simulink model "QuadCopterwhole"  (R2014b)
settings: Solver=ode23t  StartTime=0.0  StopTime=100  FixedStep=0.001  RelTol=1e-3  AbsTol=1e-4
InitFcn:
  | load SimpleDroneData
values from neighbouring files (symbols this model uses):
  m_indoorHull = 0.458    [QuadCopterParameters_m.m]
  motorCoeffs = [0.00010909388854752541 0.0075590948720063037 0.09060950915942291                 ]    [QuadCopterParameters_m.m]
libraries: simulink x2, vrlib x2, aerolibobsolete x1, aerolibtransform2 x1
settings Model: Creator=rruff  LastModifiedBy=Ehang
settings DataIOCC: SignalLoggingSaveFormat=ModelDataLogs  SaveOutput=off  SaveTime=off
settings OptimizationCC: InlineParams=on  ExpressionDepthLimit=2147483647  LifeSpan=1
settings DebuggingCC: UnderspecifiedInitializationDetection=Classic  MergeDetectMultiDrivingBlocksExec=none  SolverPrmCheckMsg=none  MultiTaskDSMMsg=warning  MultiTaskCondExecSysMsg=none  FcnCallInpInsideContextMsg=EnableAllAsWarning  StateNameClashWarn=warning
settings HardwareCC: ProdBitPerInt=16  ProdBitPerPointer=8  ProdIntDivRoundTo=Zero  ProdEndianess=LittleEndian  ProdWordSize=8  ProdHWDeviceType=Atmel->AVR
settings RTWCC: IncludeERTFirstTime=on
settings SimscapeCC: SelectedTab=SimMechanics2G
settings SimMechanicsCC: VisOnUpdateDiagram=on  VisDuringSimulation=on  FramesToBeSkipped=10  AnimationDelay=0  LastVizWinPosition=[1022 659 560 420]  CamPosition=[10.2752;-3.21889;-2.95529;]  CamTarget=[0;-2.23517e-09;-0.0242675;]  CamUpVector=[-0.23308;0.133123;-0.963303;]  CamHeight=0.224542  VisBackgroundColor=[0.9;0.9;0.95;]  DefaultBodyColor=[1;0;0;]
settings ExplorerConfigSet: SimMechanicsOpenEditorOnUpdate=off

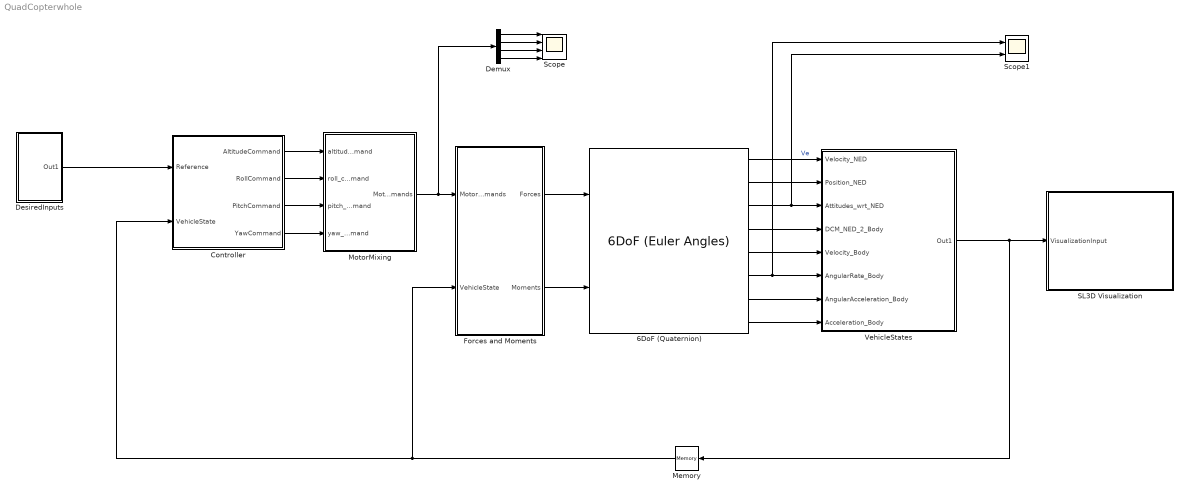
== system QuadCopterwhole ==
  6DoF (Quaternion) : aerolibobsolete/6DoF (Euler Angles)  units=Metric (MKS)  mtype=Fixed  rep=Quaternion  xme_0=[0 0 0]  Vm_0=[0 0 0]  eul_0=[0 0 0]  pm_0=[0 0 0]  mass_0=Mass  mass_e=0  mass_f=0  inertia=MomentInertiaTensor  inertia_e=eye(3)  inertia_f=eye(3)  k_quat=1.0
  Controller : Subsystem
  Demux : Demux
  DesiredInputs : Subsystem
  Forces and Moments : Subsystem  TreatAsAtomicUnit=on
  Memory : Memory
  MotorMixing : Subsystem
  SL3D Visualization : Subsystem
  Scope : Scope  NumInputPorts=4
      settings: YMin=-5~-5~-5~-5  YMax=5~5~5~5
  Scope1 : Scope  NumInputPorts=2
      settings: YMin=-5~-5  YMax=5~5  SaveName=ScopeData5
  VehicleStates : Subsystem
  wires:
  Forces and Moments/1(Forces) -> 6DoF (Quaternion)/1
  Forces and Moments/2(Moments) -> 6DoF (Quaternion)/2
  6DoF (Quaternion)/6 -> Scope1/1, VehicleStates/6(AngularRate_Body)
  6DoF (Quaternion)/8 -> VehicleStates/8(Acceleration_Body)
  6DoF (Quaternion)/4 -> VehicleStates/4(DCM_NED_2_Body)
  6DoF (Quaternion)/5 -> VehicleStates/5(Velocity_Body)
  6DoF (Quaternion)/7 -> VehicleStates/7(AngularAcceleration_Body)
  6DoF (Quaternion)/3 -> Scope1/2, VehicleStates/3(Attitudes_wrt_NED)
  6DoF (Quaternion)/2 -> VehicleStates/2(Position_NED)
  6DoF (Quaternion)/1 -> VehicleStates/1(Velocity_NED)  "Ve"
  Controller/1(AltitudeCommand) -> MotorMixing/1(altitude_command)
  Controller/2(RollCommand) -> MotorMixing/2(roll_command)
  Controller/3(PitchCommand) -> MotorMixing/3(pitch_command)
  MotorMixing/1(MotorCommands) -> Demux/1, Forces and Moments/1(MotorCommands)
  Controller/4(YawCommand) -> MotorMixing/4(yaw_command)
  Memory/1 -> Controller/2(VehicleState), Forces and Moments/2(VehicleState)
  VehicleStates/1(Out1) -> SL3D Visualization/1(VisualizationInput), Memory/1
  DesiredInputs/1(Out1) -> Controller/1(Reference)
  Demux/2 -> Scope/2
  Demux/1 -> Scope/1
  Demux/3 -> Scope/3
  Demux/4 -> Scope/4

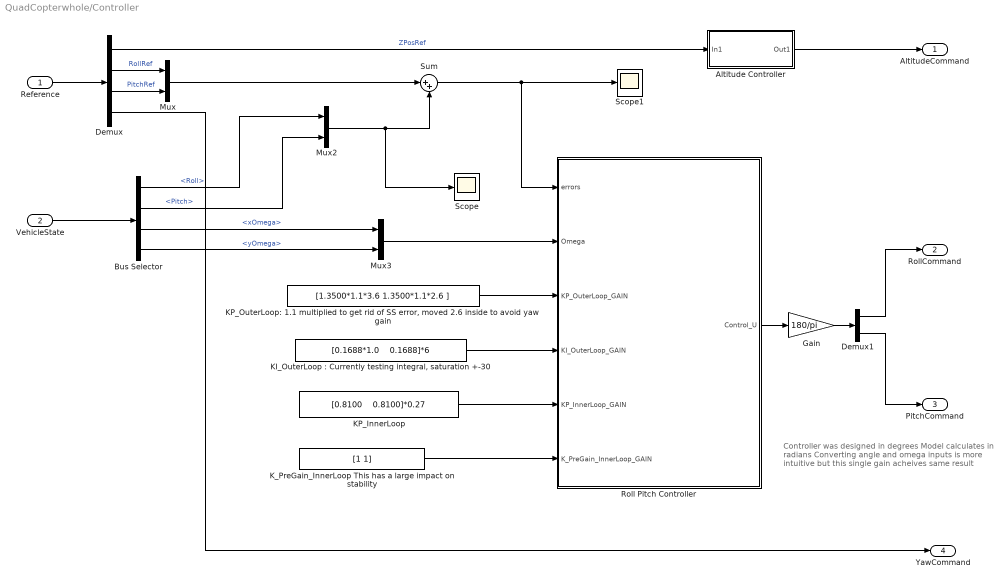
== system QuadCopterwhole/Controller ==
  note: Controller was designed in degrees
      | Model calculates in radians
      | Converting angle and omega inputs is more
      | intuitive but this single gain acheives same result
  Reference : Inport
  VehicleState : Inport  Port=2
  Altitude Controller : Subsystem
  Bus Selector : BusSelector  OutputSignals=NEDState.Attitude.Roll,NEDState.Attitude.Pitch,BodyState.AngularRate.xOmega,BodyState.AngularRate.yOmega
  Demux : Demux
  Demux1 : Demux  Outputs=2
  Gain : Gain  Gain=180/pi
  "KI_OuterLoop : Currently testing integral, saturation +-30" : Constant  Value="[0.1688*1.0    0.1688]*6"
  KP_InnerLoop : Constant  Value="[0.8100    0.8100]*0.27"
  "KP_OuterLoop: 1.1 multiplied to get rid of SS error, moved 2.6 inside to avoid yaw gain" : Constant  Value=[1.3500*1.1*3.6 1.3500*1.1*2.6 ]
  K_PreGain_InnerLoop This has a large impact on stability : Constant  Value=[1 1]
  Mux : Mux  Inputs=2
  Mux2 : Mux  Inputs=2
  Mux3 : Mux  Inputs=2
  Roll Pitch Controller : Subsystem  TreatAsAtomicUnit=on
  Scope : Scope
      settings: SaveName=ScopeData3
  Scope1 : Scope
      settings: SaveName=ScopeData11
  Sum : Sum  Inputs=|++
  AltitudeCommand : Outport
  RollCommand : Outport  Port=2
  PitchCommand : Outport  Port=3
  YawCommand : Outport  Port=4
  wires:
  Reference/1 -> Demux/1
  VehicleState/1 -> Bus Selector/1
  Demux/1 -> Altitude Controller/1(In1)  "ZPosRef"
  Demux/3 -> Mux/2  "PitchRef"
  Demux/2 -> Mux/1  "RollRef"
  Mux/1 -> Sum/1
  Mux2/1 -> Scope/1, Sum/2
  Sum/1 -> Scope1/1, Roll Pitch Controller/1(errors)
  Bus Selector/1 -> Mux2/1  "<Roll>"
  Bus Selector/2 -> Mux2/2  "<Pitch>"
  Bus Selector/3 -> Mux3/1  "<xOmega>"
  Bus Selector/4 -> Mux3/2  "<yOmega>"
  Mux3/1 -> Roll Pitch Controller/2(Omega)
  "KP_OuterLoop: 1.1 multiplied to get rid of SS error, moved 2.6 inside to avoid yaw gain"/1 -> Roll Pitch Controller/3(KP_OuterLoop_GAIN)
  K_PreGain_InnerLoop This has a large impact on stability/1 -> Roll Pitch Controller/6(K_PreGain_InnerLoop_GAIN)
  KP_InnerLoop/1 -> Roll Pitch Controller/5(KP_InnerLoop_GAIN)
  "KI_OuterLoop : Currently testing integral, saturation +-30"/1 -> Roll Pitch Controller/4(KI_OuterLoop_GAIN)
  Roll Pitch Controller/1(Control_U) -> Gain/1
  Demux1/1 -> RollCommand/1
  Demux1/2 -> PitchCommand/1
  Demux/4 -> YawCommand/1
  Gain/1 -> Demux1/1
  Altitude Controller/1(Out1) -> AltitudeCommand/1

== system QuadCopterwhole/DesiredInputs ==
  Mux : Mux
  Step : Step  Time=3  After=-1  SampleTime=0
  Step1 : Step  Time=2  After=0  SampleTime=0
  Step2 : Step  Time=5  After=0  SampleTime=0
  Step3 : Step  Time=5  After=0  SampleTime=0
  Out1 : Outport
  wires:
  Step1/1 -> Mux/2  "RollRef"
  Step/1 -> Mux/1  "ZPosRef"
  Step2/1 -> Mux/3  "PitchRef"
  Mux/1 -> Out1/1  "Reference"
  Step3/1 -> Mux/4  "YawRef"

== system QuadCopterwhole/Forces and Moments ==
  MotorCommands : Inport
  VehicleState : Inport  Port=2
  Applied Force Calculation : Subsystem
  Applied torque Calculation1 : Subsystem
  Display : Display
  Gravity Force Calculation : Subsystem
  Motor Forces and Torques : Subsystem
  Scope : Scope
      settings: SaveName=ScopeData4
  Forces : Outport
  Moments : Outport  Port=2
  wires:
  Motor Forces and Torques/1(Motor Forces) -> Applied torque Calculation1/1(Motor Forces), Applied Force Calculation/2(Motor Forces)
  Applied Force Calculation/1(External Forces) -> Forces/1
  Motor Forces and Torques/2(Motor Torques) -> Applied torque Calculation1/2(Motor Torques)
  Applied torque Calculation1/1(External Torques) -> Display/1, Moments/1
  MotorCommands/1 -> Motor Forces and Torques/1(Motor Commands)
  VehicleState/1 -> Gravity Force Calculation/1(posinfo)
  Gravity Force Calculation/1(gravity force) -> Scope/1, Applied Force Calculation/1(gravity force)

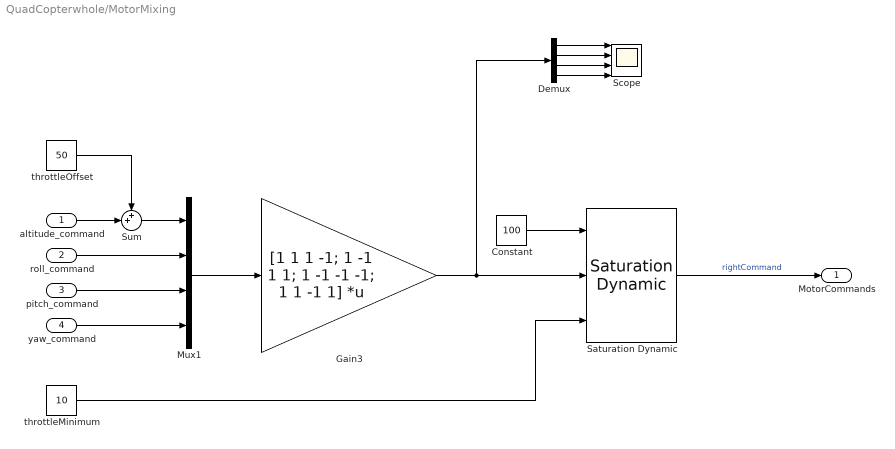
== system QuadCopterwhole/MotorMixing ==
  altitude_command : Inport
  roll_command : Inport  Port=2
  pitch_command : Inport  Port=3
  yaw_command : Inport  Port=4
  Constant : Constant  Value=100
  Demux : Demux
  Gain3 : Gain  Gain=[1 1 1 -1; 1 -1 1 1; 1 -1 -1 -1; 1 1 -1 1]  Multiplication=Matrix(K*u)  ParamDataTypeStr=int16
  Mux1 : Mux
  Saturation Dynamic : simulink/Discontinuities/Saturation Dynamic  OutMin=[]  OutMax=[]  OutDataTypeStr=Inherit: Same as second input  OutDataType=fixdt(1, 16)  OutScaling=2^-10  DoSatur=off
  Scope : Scope  NumInputPorts=4
      settings: TimeRange=100  YMin=-5~-5~-5~-5  YMax=5~5~5~5  SaveName=ScopeData2
  Sum : Sum  Inputs=++|
  throttleMinimum : Constant  Value=10
  throttleOffset : Constant  Value=50
  MotorCommands : Outport
  wires:
  yaw_command/1 -> Mux1/4
  pitch_command/1 -> Mux1/3
  roll_command/1 -> Mux1/2
  Mux1/1 -> Gain3/1
  altitude_command/1 -> Sum/2
  Sum/1 -> Mux1/1
  throttleOffset/1 -> Sum/1
  throttleMinimum/1 -> Saturation Dynamic/3
  Constant/1 -> Saturation Dynamic/1
  Saturation Dynamic/1 -> MotorCommands/1  "rightCommand"
  Gain3/1 -> Demux/1, Saturation Dynamic/2
  Demux/2 -> Scope/2
  Demux/1 -> Scope/1
  Demux/3 -> Scope/3
  Demux/4 -> Scope/4

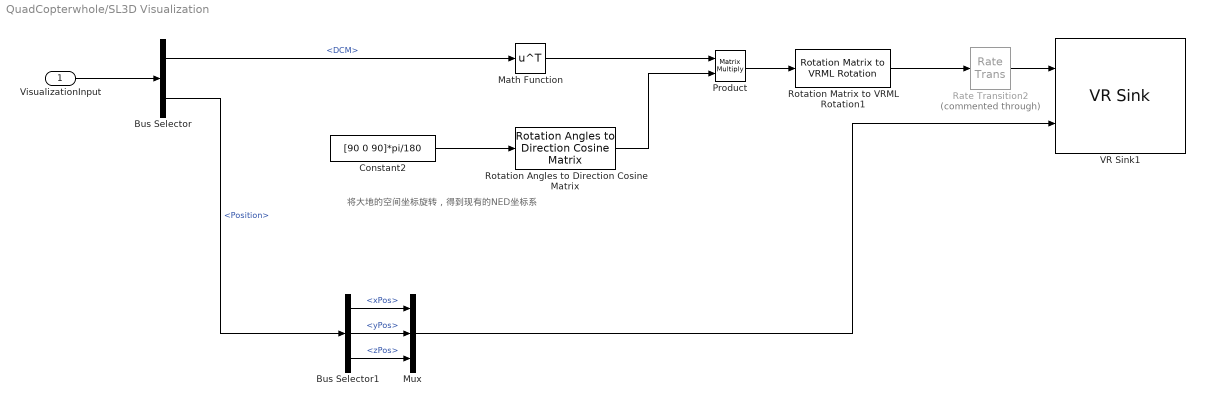
== system QuadCopterwhole/SL3D Visualization ==
  note: 将大地的空间坐标旋转，得到现有的NED坐标系
  VisualizationInput : Inport
  Bus Selector : BusSelector  OutputSignals=NEDState.Attitude.DCM,NEDState.Position
  Bus Selector1 : BusSelector  OutputSignals=xPos,yPos,zPos
  Constant2 : Constant  Value=[90 0 90]*pi/180
  Math Function : Math  Operator=transpose  SaturateOnIntegerOverflow=on
  Mux : Mux  Inputs=3
  Product : Product  Multiplication=Matrix(*)
  Rate Transition2 : RateTransition  Commented=through
  Rotation Angles to Direction Cosine Matrix : aerolibtransform2/Rotation Angles to Direction Cosine Matrix  rotationOrder=XYZ
  Rotation Matrix to VRML Rotation1 : vrlib/Utilities/Rotation Matrix to VRML Rotation  maxzero=1e-12
  VR Sink1 : vrlib/VR Sink  InstantiateOnLoad=on  SampleTime=-1  ViewEnable=on  RemoteChange=off  RemoteView=off  FieldsWritten=Drone.rotation.4.1.1.double#Drone.translation.3.1.1.double  WorldFileName=myDrone3.wrl  AutoView=off  VideoDimensions=[]  AllowVariableSize=off
  wires:
  VisualizationInput/1 -> Bus Selector/1
  Rotation Matrix to VRML Rotation1/1 -> Rate Transition2/1
  Rate Transition2/1 -> VR Sink1/1
  Bus Selector/2 -> Bus Selector1/1  "<Position>"
  Mux/1 -> VR Sink1/2
  Constant2/1 -> Rotation Angles to Direction Cosine Matrix/1
  Rotation Angles to Direction Cosine Matrix/1 -> Product/2
  Math Function/1 -> Product/1
  Product/1 -> Rotation Matrix to VRML Rotation1/1
  Bus Selector/1 -> Math Function/1  "<DCM>"
  Bus Selector1/1 -> Mux/1  "<xPos>"
  Bus Selector1/2 -> Mux/2  "<yPos>"
  Bus Selector1/3 -> Mux/3  "<zPos>"

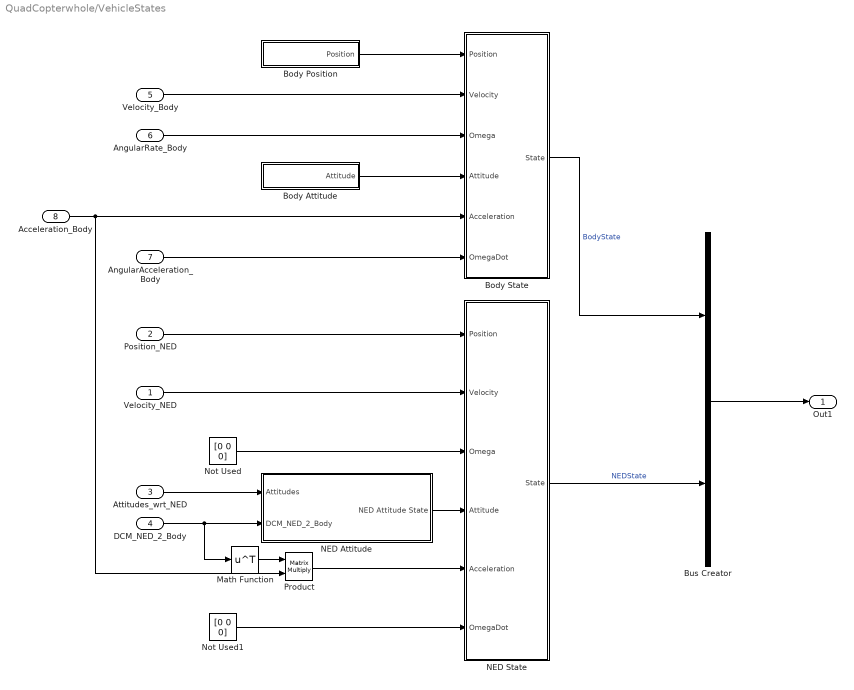
== system QuadCopterwhole/VehicleStates ==
  Velocity_NED : Inport
  Position_NED : Inport  Port=2
  Attitudes_wrt_NED : Inport  Port=3
  DCM_NED_2_Body : Inport  Port=4
  Velocity_Body : Inport  Port=5
  AngularRate_Body : Inport  Port=6
  AngularAcceleration_Body : Inport  Port=7
  Acceleration_Body : Inport  Port=8
  Body Attitude : Subsystem
  Body Position : Subsystem
  Body State : Subsystem
  Bus Creator : BusCreator  Inputs=2  OutDataTypeStr=Bus: VehicleStates  NonVirtualBus=on
  Math Function : Math  Operator=transpose  SaturateOnIntegerOverflow=on
  NED Attitude : Subsystem
  NED State : Subsystem
  Not Used : Constant  Value=[0 0 0]
  Not Used1 : Constant  Value=[0 0 0]
  Product : Product  Multiplication=Matrix(*)
  Out1 : Outport
  wires:
  Bus Creator/1 -> Out1/1
  Velocity_NED/1 -> NED State/2(Velocity)
  NED Attitude/1(NED Attitude State) -> NED State/4(Attitude)
  Position_NED/1 -> NED State/1(Position)
  Attitudes_wrt_NED/1 -> NED Attitude/1(Attitudes)
  NED State/1(State) -> Bus Creator/2  "NEDState"
  Body State/1(State) -> Bus Creator/1  "BodyState"
  Body Attitude/1(Attitude) -> Body State/4(Attitude)
  DCM_NED_2_Body/1 -> Math Function/1, NED Attitude/2(DCM_NED_2_Body)
  Acceleration_Body/1 -> Product/2, Body State/5(Acceleration)
  AngularAcceleration_Body/1 -> Body State/6(OmegaDot)
  Velocity_Body/1 -> Body State/2(Velocity)
  Body Position/1(Position) -> Body State/1(Position)
  AngularRate_Body/1 -> Body State/3(Omega)
  Not Used/1 -> NED State/3(Omega)
  Not Used1/1 -> NED State/6(OmegaDot)
  Product/1 -> NED State/5(Acceleration)
  Math Function/1 -> Product/1

== system QuadCopterwhole/Controller/Altitude Controller ==
  In1 : Inport
  Out1 : Outport
  wires:
  In1/1 -> Out1/1

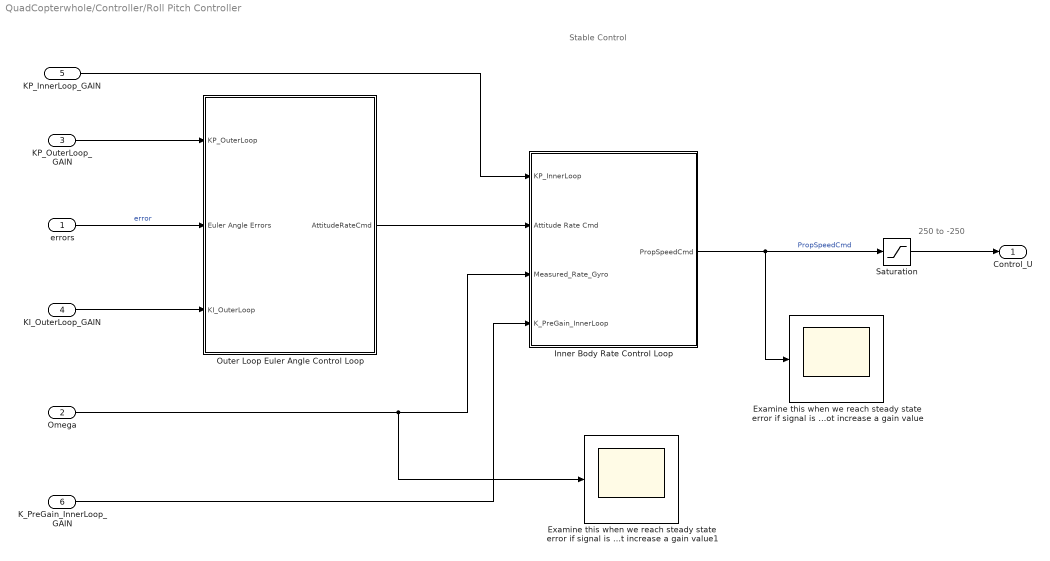
== system QuadCopterwhole/Controller/Roll Pitch Controller ==
  note: 250 to -250
  note: Stable Control
  errors : Inport
  Omega : Inport  Port=2
  KP_OuterLoop_GAIN : Inport  Port=3
  KI_OuterLoop_GAIN : Inport  Port=4
  KP_InnerLoop_GAIN : Inport  Port=5
  K_PreGain_InnerLoop_GAIN : Inport  Port=6
  Examine this when we reach steady state error if signal is abs(0)<1 then we need ot increase a gain value : Scope
      settings: YMin=-6  YMax=4  SaveName=ScopeData7
  Examine this when we reach steady state error if signal is abs(0)<1 then we need ot increase a gain value1 : Scope
      settings: YMin=-3.62958e-15  YMax=40
  Inner Body Rate Control Loop : Subsystem
  Outer Loop Euler Angle Control Loop : Subsystem
  Saturation : Saturate  UpperLimit=250  LowerLimit=-250  OutDataTypeStr=Inherit: Inherit via back propagation
      settings: AttributesFormatString=%<LowerLimit>\nto\n%<UpperLimit>
  Control_U : Outport
  wires:
  Saturation/1 -> Control_U/1
  KP_InnerLoop_GAIN/1 -> Inner Body Rate Control Loop/1(KP_InnerLoop)
  Omega/1 -> Examine this when we reach steady state error if signal is abs(0)<1 then we need ot increase a gain value1/1, Inner Body Rate Control Loop/3(Measured_Rate_Gyro)
  K_PreGain_InnerLoop_GAIN/1 -> Inner Body Rate Control Loop/4(K_PreGain_InnerLoop)
  Inner Body Rate Control Loop/1(PropSpeedCmd) -> Saturation/1, Examine this when we reach steady state error if signal is abs(0)<1 then we need ot increase a gain value/1  "PropSpeedCmd"
  KP_OuterLoop_GAIN/1 -> Outer Loop Euler Angle Control Loop/1(KP_OuterLoop)
  errors/1 -> Outer Loop Euler Angle Control Loop/2(Euler Angle Errors)  "error"
  KI_OuterLoop_GAIN/1 -> Outer Loop Euler Angle Control Loop/3(KI_OuterLoop)
  Outer Loop Euler Angle Control Loop/1(AttitudeRateCmd) -> Inner Body Rate Control Loop/2(Attitude Rate Cmd)

== system QuadCopterwhole/Forces and Moments/Applied Force Calculation ==
  gravity force : Inport
  Motor Forces : Inport  Port=2
  Add : Sum  Inputs=+
  Add1 : Sum
  Constant : Constant  Value=[0 0]
  Mux : Mux  Inputs=2
  External Forces : Outport
  wires:
  Add/1 -> Mux/2  "Vertical Thrust"
  Constant/1 -> Mux/1
  Add1/1 -> External Forces/1
  Motor Forces/1 -> Add/1
  Mux/1 -> Add1/2  "Motor Thrust"
  gravity force/1 -> Add1/1

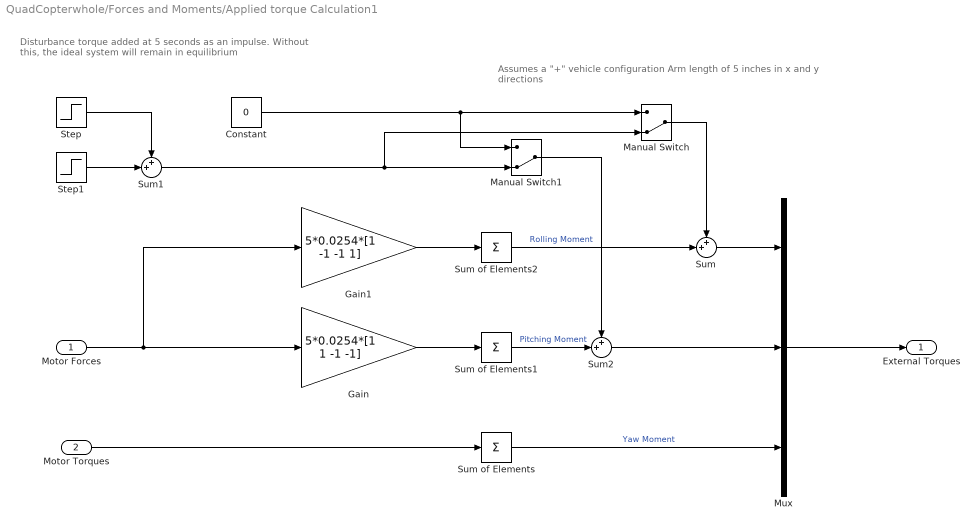
== system QuadCopterwhole/Forces and Moments/Applied torque Calculation1 ==
  note: Disturbance torque added at 5 seconds as an impulse.
      | Without this, the ideal system will remain in equilibrium
  note: Assumes a "+" vehicle configuration
      | Arm length of 5 inches in x and y directions
  Motor Forces : Inport
  Motor Torques : Inport  Port=2
  Constant : Constant  Value=0
  Gain : Gain  Gain=5*0.0254*[1 1 -1 -1]
  Gain1 : Gain  Gain=5*0.0254*[1 -1 -1 1]
  Manual Switch : ManualSwitch  CurrentSetting=0
  Manual Switch1 : ManualSwitch  CurrentSetting=0
  Mux : Mux  Inputs=3
  Step : Step  Time=5  SampleTime=0
  Step1 : Step  Time=5.01  After=-1  SampleTime=0
  Sum : Sum  Inputs=++|
  Sum of Elements : Sum  Inputs=+
  Sum of Elements1 : Sum  Inputs=+
  Sum of Elements2 : Sum  Inputs=+
  Sum1 : Sum  Inputs=++|
  Sum2 : Sum  Inputs=++|
  External Torques : Outport
  wires:
  Motor Torques/1 -> Sum of Elements/1
  Sum of Elements/1 -> Mux/3  "Yaw Moment"
  Motor Forces/1 -> Gain/1, Gain1/1
  Gain/1 -> Sum of Elements1/1
  Gain1/1 -> Sum of Elements2/1
  Mux/1 -> External Torques/1
  Sum/1 -> Mux/1
  Sum of Elements2/1 -> Sum/2  "Rolling Moment"
  Step1/1 -> Sum1/2
  Step/1 -> Sum1/1
  Sum2/1 -> Mux/2
  Sum of Elements1/1 -> Sum2/2  "Pitching Moment"
  Constant/1 -> Manual Switch1/1, Manual Switch/1
  Manual Switch/1 -> Sum/1
  Manual Switch1/1 -> Sum2/1
  Sum1/1 -> Manual Switch/2, Manual Switch1/2

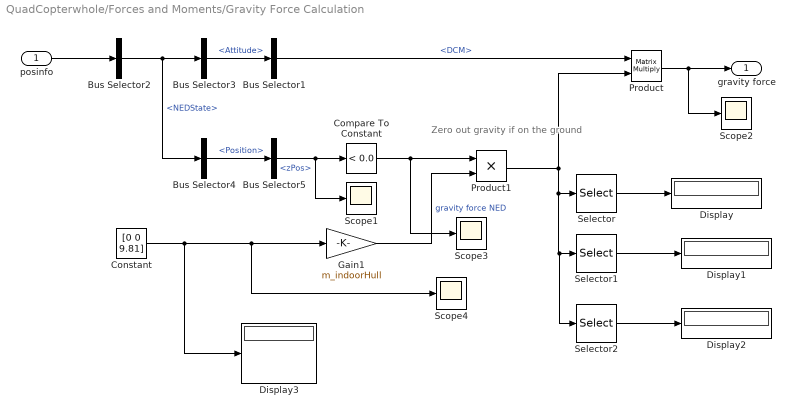
== system QuadCopterwhole/Forces and Moments/Gravity Force Calculation ==
  note: Zero out gravity if on the ground
  posinfo : Inport
  Bus Selector1 : BusSelector  OutputSignals=DCM
  Bus Selector2 : BusSelector  OutputSignals=NEDState
  Bus Selector3 : BusSelector  OutputSignals=Attitude
  Bus Selector4 : BusSelector  OutputSignals=Position
  Bus Selector5 : BusSelector  OutputSignals=zPos
  Compare To Constant : simulink/Logic and Bit Operations/Compare To Constant  relop=<  const=0.0  OutDataTypeStr=boolean
  Constant : Constant  Value=[0 0 9.81]
  Display{,1..3} (4 alike) : Display
  Gain1 : Gain  Gain=m_indoorHull
  Product : Product  Multiplication=Matrix(*)
  Product1 : Product
  Scope{1..4} (4 alike) : Scope
      Scope1 settings: SaveName=ScopeData8
      Scope2 settings: SaveName=ScopeData7
      Scope3 settings: SaveName=ScopeData9
      Scope4 settings: SaveName=ScopeData10
  Selector : Selector  InputPortWidth=3  Indices=[1]
  Selector1 : Selector  InputPortWidth=3  Indices=[2]
  Selector2 : Selector  InputPortWidth=3  Indices=[3]
  gravity force : Outport
  wires:
  Bus Selector3/1 -> Bus Selector1/1  "<Attitude>"
  Bus Selector2/1 -> Bus Selector4/1, Bus Selector3/1  "<NEDState>"
  posinfo/1 -> Bus Selector2/1
  Bus Selector1/1 -> Product/1  "<DCM>"
  Constant/1 -> Display3/1, Scope4/1, Gain1/1
  Gain1/1 -> Product1/2  "gravity force NED"
  Product/1 -> Scope2/1, gravity force/1
  Bus Selector4/1 -> Bus Selector5/1  "<Position>"
  Bus Selector5/1 -> Scope1/1, Compare To Constant/1  "<zPos>"
  Product1/1 -> Product/2, Selector2/1, Selector1/1, Selector/1
  Compare To Constant/1 -> Scope3/1, Product1/1
  Selector/1 -> Display/1
  Selector1/1 -> Display1/1
  Selector2/1 -> Display2/1

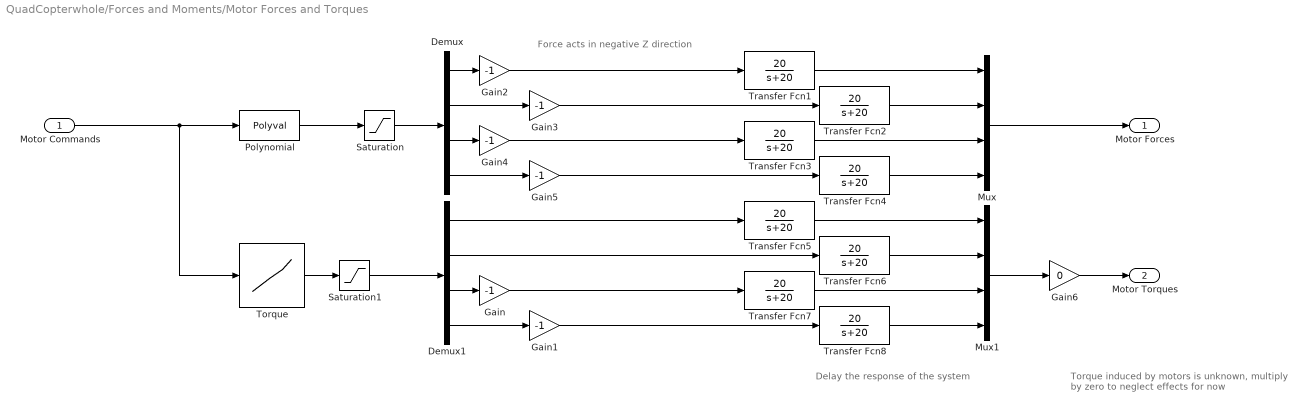
== system QuadCopterwhole/Forces and Moments/Motor Forces and Torques ==
  note: Force acts in negative Z direction
  note: Delay the response of the system
  note: Torque induced by motors is unknown,
      | multiply by zero to neglect effects for now
  Motor Commands : Inport
  Demux : Demux
  Demux1 : Demux
  Gain{,1..5} (6 alike) : Gain  Gain=-1
  Gain6 : Gain  Gain=0
  Mux : Mux
  Mux1 : Mux
  Polynomial : Polyval  Coefs=motorCoeffs
  Saturation : Saturate  UpperLimit=8.1  LowerLimit=0
  Saturation1 : Saturate  UpperLimit=0.189  LowerLimit=0
  Torque : Lookup_n-D  NumberOfTableDimensions=1  BreakpointsForDimension1="[1160  1300  1389  1500   1600  1720  1824]"  Table="0.00980665*0.3048*[0        10    20    35     42    58    63]"  ExtrapMethod=Clip  UseLastTableValue=on  RndMeth=Simplest  InputSameDT=on
  Transfer Fcn{1..8} (8 alike) : TransferFcn  Numerator=[20]  Denominator=[1 20]
  Motor Forces : Outport
  Motor Torques : Outport  Port=2
  wires:
  Transfer Fcn8/1 -> Mux1/4
  Transfer Fcn3/1 -> Mux/3
  Transfer Fcn5/1 -> Mux1/1
  Gain/1 -> Transfer Fcn7/1
  Saturation1/1 -> Demux1/1
  Transfer Fcn6/1 -> Mux1/2
  Transfer Fcn1/1 -> Mux/1
  Gain5/1 -> Transfer Fcn4/1
  Transfer Fcn4/1 -> Mux/4
  Gain1/1 -> Transfer Fcn8/1
  Transfer Fcn7/1 -> Mux1/3
  Transfer Fcn2/1 -> Mux/2
  Saturation/1 -> Demux/1
  Gain4/1 -> Transfer Fcn3/1
  Gain3/1 -> Transfer Fcn2/1
  Gain2/1 -> Transfer Fcn1/1
  Demux1/4 -> Gain1/1
  Demux1/3 -> Gain/1
  Demux1/2 -> Transfer Fcn6/1
  Demux1/1 -> Transfer Fcn5/1
  Torque/1 -> Saturation1/1
  Demux/4 -> Gain5/1
  Demux/3 -> Gain4/1
  Demux/2 -> Gain3/1
  Demux/1 -> Gain2/1
  Polynomial/1 -> Saturation/1
  Mux/1 -> Motor Forces/1
  Mux1/1 -> Gain6/1
  Motor Commands/1 -> Polynomial/1, Torque/1
  Gain6/1 -> Motor Torques/1

== system QuadCopterwhole/VehicleStates/Body Attitude ==
  Bus Creator1 : BusCreator  OutDataTypeStr=Bus: AttitudeBus  NonVirtualBus=on
  Constant : Constant  Value=0
  Constant1 : Constant  Value=0
  Constant2 : Constant  Value=0
  Constant3 : Constant  Value=eye(3)
  Attitude : Outport
  wires:
  Constant/1 -> Bus Creator1/1  "Roll"
  Bus Creator1/1 -> Attitude/1
  Constant1/1 -> Bus Creator1/2  "Pitch"
  Constant2/1 -> Bus Creator1/3  "Yaw"
  Constant3/1 -> Bus Creator1/4  "DCM"

== system QuadCopterwhole/VehicleStates/Body Position ==
  Constant : Constant  Value=0
  Constant1 : Constant  Value=0
  Constant2 : Constant  Value=0
  Mux : Mux  Inputs=3
  Position : Outport
  wires:
  Constant2/1 -> Mux/3  "Z"
  Constant1/1 -> Mux/2  "Y"
  Constant/1 -> Mux/1  "X"
  Mux/1 -> Position/1

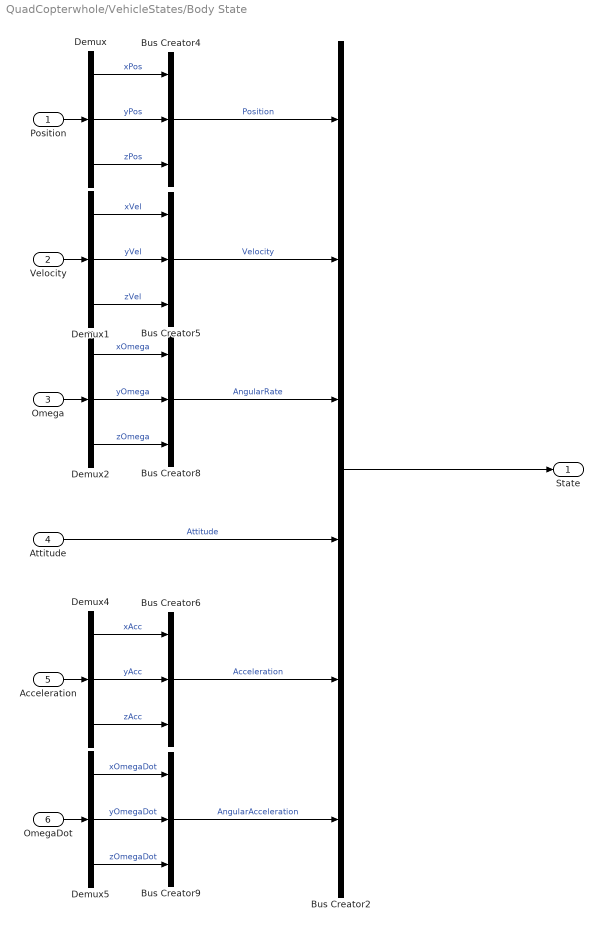
== system QuadCopterwhole/VehicleStates/Body State ==
  Position : Inport
  Velocity : Inport  Port=2
  Omega : Inport  Port=3
  Attitude : Inport  Port=4
  Acceleration : Inport  Port=5
  OmegaDot : Inport  Port=6
  Bus Creator2 : BusCreator  Inputs=6  OutDataTypeStr=Bus: States  NonVirtualBus=on
  Bus Creator4 : BusCreator  Inputs=3  OutDataTypeStr=Bus: PositionBus  NonVirtualBus=on
  Bus Creator5 : BusCreator  Inputs=3  OutDataTypeStr=Bus: VelocityBus  NonVirtualBus=on
  Bus Creator6 : BusCreator  Inputs=3  OutDataTypeStr=Bus: AccelerationBus  NonVirtualBus=on
  Bus Creator8 : BusCreator  Inputs=3  OutDataTypeStr=Bus: AngularRateBus  NonVirtualBus=on
  Bus Creator9 : BusCreator  Inputs=3  OutDataTypeStr=Bus: AngularAccelerationBus  NonVirtualBus=on
  Demux{,1..2,4..5} (5 alike) : Demux  Outputs=3
  State : Outport  OutDataTypeStr=Bus: States
  wires:
  Demux/1 -> Bus Creator4/1  "xPos"
  Demux/2 -> Bus Creator4/2  "yPos"
  Demux/3 -> Bus Creator4/3  "zPos"
  Demux1/1 -> Bus Creator5/1  "xVel"
  Demux1/2 -> Bus Creator5/2  "yVel"
  Demux1/3 -> Bus Creator5/3  "zVel"
  Demux2/1 -> Bus Creator8/1  "xOmega"
  Demux2/2 -> Bus Creator8/2  "yOmega"
  Demux2/3 -> Bus Creator8/3  "zOmega"
  Demux4/1 -> Bus Creator6/1  "xAcc"
  Demux4/2 -> Bus Creator6/2  "yAcc"
  Demux4/3 -> Bus Creator6/3  "zAcc"
  Demux5/1 -> Bus Creator9/1  "xOmegaDot"
  Demux5/2 -> Bus Creator9/2  "yOmegaDot"
  Demux5/3 -> Bus Creator9/3  "zOmegaDot"
  Bus Creator4/1 -> Bus Creator2/1  "Position"
  Bus Creator5/1 -> Bus Creator2/2  "Velocity"
  Bus Creator8/1 -> Bus Creator2/3  "AngularRate"
  Attitude/1 -> Bus Creator2/4  "Attitude"
  Bus Creator6/1 -> Bus Creator2/5  "Acceleration"
  Bus Creator9/1 -> Bus Creator2/6  "AngularAcceleration"
  Position/1 -> Demux/1
  Velocity/1 -> Demux1/1
  Omega/1 -> Demux2/1
  Bus Creator2/1 -> State/1
  Acceleration/1 -> Demux4/1
  OmegaDot/1 -> Demux5/1

== system QuadCopterwhole/VehicleStates/NED Attitude ==
  Attitudes : Inport
  DCM_NED_2_Body : Inport  Port=2
  Bus Creator7 : BusCreator  OutDataTypeStr=Bus: AttitudeBus  NonVirtualBus=on
  Demux3 : Demux  Outputs=3
  NED Attitude State : Outport
  wires:
  Attitudes/1 -> Demux3/1
  DCM_NED_2_Body/1 -> Bus Creator7/4  "DCM"
  Demux3/1 -> Bus Creator7/1  "Roll"
  Bus Creator7/1 -> NED Attitude State/1  "Attitude"
  Demux3/3 -> Bus Creator7/3  "Yaw"
  Demux3/2 -> Bus Creator7/2  "Pitch"

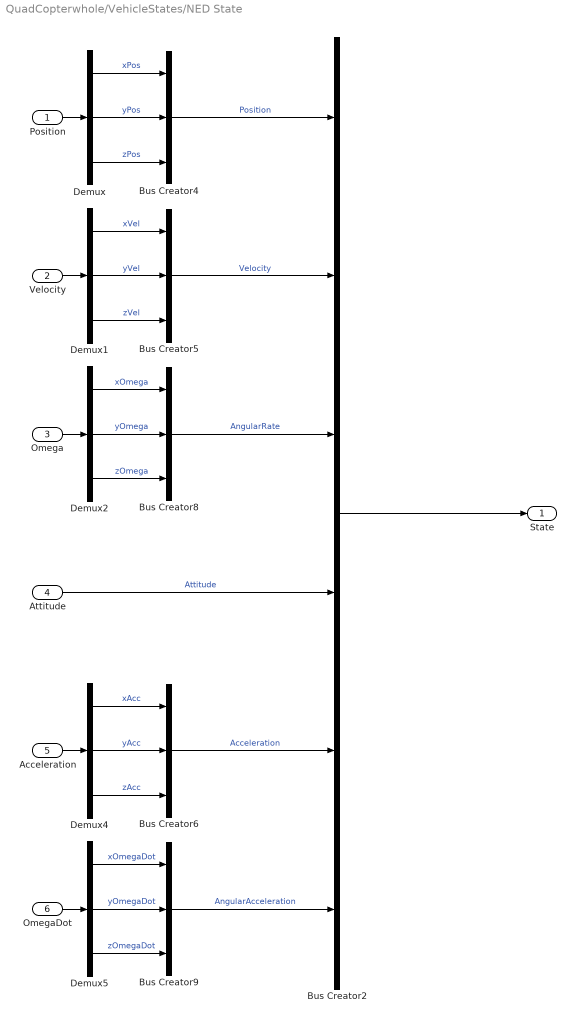
== system QuadCopterwhole/VehicleStates/NED State ==
  Position : Inport
  Velocity : Inport  Port=2
  Omega : Inport  Port=3
  Attitude : Inport  Port=4
  Acceleration : Inport  Port=5
  OmegaDot : Inport  Port=6
  Bus Creator2 : BusCreator  Inputs=6  OutDataTypeStr=Bus: States  NonVirtualBus=on
  Bus Creator4 : BusCreator  Inputs=3  OutDataTypeStr=Bus: PositionBus  NonVirtualBus=on
  Bus Creator5 : BusCreator  Inputs=3  OutDataTypeStr=Bus: VelocityBus  NonVirtualBus=on
  Bus Creator6 : BusCreator  Inputs=3  OutDataTypeStr=Bus: AccelerationBus  NonVirtualBus=on
  Bus Creator8 : BusCreator  Inputs=3  OutDataTypeStr=Bus: AngularRateBus  NonVirtualBus=on
  Bus Creator9 : BusCreator  Inputs=3  OutDataTypeStr=Bus: AngularAccelerationBus  NonVirtualBus=on
  Demux{,1..2,4..5} (5 alike) : Demux  Outputs=3
  State : Outport  OutDataTypeStr=Bus: States
  wires:
  Demux/1 -> Bus Creator4/1  "xPos"
  Demux/2 -> Bus Creator4/2  "yPos"
  Demux/3 -> Bus Creator4/3  "zPos"
  Demux1/1 -> Bus Creator5/1  "xVel"
  Demux1/2 -> Bus Creator5/2  "yVel"
  Demux1/3 -> Bus Creator5/3  "zVel"
  Demux2/1 -> Bus Creator8/1  "xOmega"
  Demux2/2 -> Bus Creator8/2  "yOmega"
  Demux2/3 -> Bus Creator8/3  "zOmega"
  Demux4/1 -> Bus Creator6/1  "xAcc"
  Demux4/2 -> Bus Creator6/2  "yAcc"
  Demux4/3 -> Bus Creator6/3  "zAcc"
  Demux5/1 -> Bus Creator9/1  "xOmegaDot"
  Demux5/2 -> Bus Creator9/2  "yOmegaDot"
  Demux5/3 -> Bus Creator9/3  "zOmegaDot"
  Bus Creator4/1 -> Bus Creator2/1  "Position"
  Bus Creator5/1 -> Bus Creator2/2  "Velocity"
  Bus Creator8/1 -> Bus Creator2/3  "AngularRate"
  Bus Creator6/1 -> Bus Creator2/5  "Acceleration"
  Bus Creator9/1 -> Bus Creator2/6  "AngularAcceleration"
  Position/1 -> Demux/1
  Velocity/1 -> Demux1/1
  Omega/1 -> Demux2/1
  Bus Creator2/1 -> State/1
  Attitude/1 -> Bus Creator2/4  "Attitude"
  Acceleration/1 -> Demux4/1
  OmegaDot/1 -> Demux5/1

== system QuadCopterwhole/Controller/Roll Pitch Controller/Inner Body Rate Control Loop ==
  KP_InnerLoop : Inport
  Attitude Rate Cmd : Inport  Port=2
  Measured_Rate_Gyro : Inport  Port=3
  K_PreGain_InnerLoop : Inport  Port=4
  Add3 : Sum
  Product4 : Product  RndMeth=Zero
  Proportional Control : Product  RndMeth=Zero
  PropSpeedCmd : Outport
  wires:
  K_PreGain_InnerLoop/1 -> Product4/2
  Attitude Rate Cmd/1 -> Add3/1  "attitude_cmd"
  Add3/1 -> Proportional Control/2  "attitude_rate_error"
  Product4/1 -> Add3/2
  Proportional Control/1 -> PropSpeedCmd/1  "PropSpeedCmd"
  Measured_Rate_Gyro/1 -> Product4/1
  KP_InnerLoop/1 -> Proportional Control/1

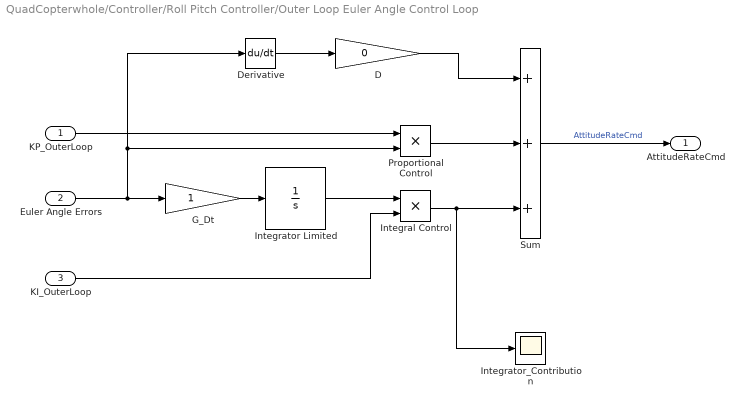
== system QuadCopterwhole/Controller/Roll Pitch Controller/Outer Loop Euler Angle Control Loop ==
  KP_OuterLoop : Inport
  Euler Angle Errors : Inport  Port=2
  KI_OuterLoop : Inport  Port=3
  D : Gain  Gain=0
  Derivative : Derivative
  G_Dt : Gain  OutDataTypeStr=double
  Integral Control : Product  RndMeth=Zero
  Integrator Limited : Integrator  LimitOutput=on  UpperSaturationLimit=[30 30]  LowerSaturationLimit=[-30 -30]
  Integrator_Contribution : Scope
      settings: YMin=0  YMax=37.5  SaveName=ScopeData6
  Proportional Control : Product  RndMeth=Zero
  Sum : Sum  Inputs=+++
  AttitudeRateCmd : Outport
  wires:
  Sum/1 -> AttitudeRateCmd/1  "AttitudeRateCmd"
  KI_OuterLoop/1 -> Integral Control/2
  G_Dt/1 -> Integrator Limited/1
  Integrator Limited/1 -> Integral Control/1
  KP_OuterLoop/1 -> Proportional Control/1
  Proportional Control/1 -> Sum/2
  Integral Control/1 -> Sum/3, Integrator_Contribution/1
  Euler Angle Errors/1 -> Derivative/1, Proportional Control/2, G_Dt/1
  Derivative/1 -> D/1
  D/1 -> Sum/1
